simulink model "PCC_Calibration_Simu"  (R2015b)
settings: Solver=ode3  StartTime=0.0  StopTime=1373  FixedStep=0.01  RelTol=1e-3
model workspace: external: MAT-File params.mat (data not in the file)
undefined symbols (not defined in the file): aeroDragCoeff, airDensity, discIntervalf, discIntervals, DiscIntNeverNeededParam, FD, frontArea, G1, G2, G3, G4, G5, G6, gravity, inertialMassVeh, iterNum, lambdaRange, magnitude, massVeh, MDL, powerWeif, powerWeis, predPeriodf, predPeriods, rollingResistCoeff, terminThreshold, terminTimedis, terminVeloweif, terminVeloweis, wheelRadius, z_ACCe
libraries: simulink x16
(part 3 of 5)

== matlab function PCC_Calibration_Simu/Road_map_information1 ==
  data: u1 input; y1 output; y2 output; y3 output
function [y1,y2,y3] = fcn(u1)
%% _________________________________________________________________________________________________________________________________________________________________外界参数 模拟地图信息，需要单独设立地图接口
dis=u1;%当前距离开始的位置
p_po=[0,-2.27524037800000,-2.26950629100000,-2.87172075000000,-2.27524037800000,-2.88893122700000,-5.48585446200000,-2.26950629100000,-1.43254373800000,-0.567237483000000,-1.43254373800000,-0.584427085000000,-0.561507627000000,0.567237483000000,-0.567237483000000,0.475560430000000,-0.475560430000000,0.475560430000000,-0.567237483000000,0,0.945423264000000,1.70193492400000,0.956883999000000,1.70193492400000,0.945423264000000,1.70193492400000,1.14026128000000,1.76498914100000,1.13453057300000,0.475560430000000,-0.475560430000000,-1.13453057300000,-0.475560430000000,-1.13453057300000,-0.475560430000000,-1.13453057300000,-2.38419243000000,-1.13453057300000,-1.91976780400000,-2.88319437200000,-2.27524037800000,-2.88319437200000,-1.70193492400000,-2.88319437200000,-2.27524037800000,-3.41685336700000,-2.37272339300000,-3.34797844600000,-2.26950629100000,-2.86598398300000,-2.27524037800000,-2.88319437200000,-1.89683677500000,-2.86598398300000,-1.70193492400000,-2.84877385200000,-1.90830225200000,-2.27524037800000,-1.42108102800000,-0.567237483000000,-1.43827511400000,-0.567237483000000,0.475560430000000,1.13453057300000,1.90830225200000,1.13453057300000,1.89683677500000,1.12879987700000,1.90830225200000,1.91976780400000,2.86598398300000,1.93123343400000,3.36519671800000,2.41860011500000,3.38815488800000,1.91976780400000,2.90040502300000,3.82446784900000,2.90040502300000,1.93123343400000,2.88893122700000,1.91403501800000,2.88893122700000,1.93123343400000,0.962614381000000,0,-0.956883999000000,-1.71339917100000,-0.962614381000000,-1.62168707500000,-1.43254373800000,0,-2.26950629100000,-1.42108102800000,-2.37845790000000,-1.70193492400000,-2.38419243000000,-3.33649976600000,-2.40139616400000,-1.69620282600000,-2.40139616400000,-1.13453057300000,-0.481290208000000,-1.12879987700000,-0.475560430000000,-1.32365024300000,0,0.567237483000000,-0.567237483000000,-0.561507627000000,-1.13453057300000,-0.475560430000000,0.567237483000000,-0.956883999000000,0,-1.12879987700000,0,-0.951153627000000,0,1.14026128000000,1.90830225200000,2.84303719900000,1.90256950400000,2.86024724400000,1.90830225200000,2.38992698400000,1.70766703900000,2.38992698400000,2.27524037800000,3.37093621000000,2.37845790000000,3.35945726000000,2.38992698400000,2.27524037800000,2.87172075000000,2.28097448800000,3.32502122000000,2.40139616400000,2.26950629100000,3.42259316500000,2.37272339300000,3.42259316500000,2.83730057400000,2.82009087100000,3.42259316500000,2.28097448800000,1.14026128000000,0,-1.14026128000000,-1.91403501800000,-1.14026128000000,-1.90830225200000,-2.84877385200000,-2.26950629100000,-2.84877385200000,-2.09749399500000,-2.28097448800000,-3.42259316500000,-2.28097448800000,-3.42259316500000,-2.83730057400000,-3.42259316500000,-2.28097448800000,-3.51443465800000,-2.83730057400000,-1.91403501800000,-2.38992698400000,-1.70766703900000,-2.40713079000000,-2.40139616400000,-1.66181059200000,-1.69047074500000,-2.84877385200000,-1.91403501800000,-1.69047074500000,-2.84877385200000,-2.21216666100000,-2.84877385200000,-2.28097448800000,-1.43827511400000,-2.28097448800000,-1.43827511400000,-2.28097448800000,-1.14026128000000,0,1.14026128000000,1.91976780400000,3.38241529500000,1.92550061000000,2.38419243000000,0.956883999000000,2.41286544000000,1.44400650500000;];
s_po=[0,0.1,20.8100000000000,58.9100000000000,66.0700000000000,67.0700000000000,70.6600000000000,86.9400000000000,116.910000000000,130.660000000000,131.660000000000,145.430000000000,169.160000000000,178.170000000000,179.160000000000,181.360000000000,183.560000000000,185.970000000000,187.150000000000,223.630000000000,253.830000000000,269.630000000000,270.640000000000,275.230000000000,276.220000000000,278.620000000000,284.150000000000,290.560000000000,290.880000000000,309.290000000000,321.680000000000,328.680000000000,329.700000000000,332.080000000000,333.080000000000,337.880000000000,342.290000000000,343.480000000000,344.490000000000,354.290000000000,355.480000000000,357.480000000000,358.680000000000,360.690000000000,363.080000000000,364.070000000000,367.270000000000,368.480000000000,370.870000000000,371.890000000000,373.070000000000,374.080000000000,391.060000000000,394.660000000000,397.060000000000,399.060000000000,401.460000000000,404.890000000000,412.690000000000,422.090000000000,428.700000000000,429.900000000000,445.490000000000,462.270000000000,476.060000000000,477.270000000000,481.670000000000,484.050000000000,485.060000000000,492.870000000000,497.630000000000,503.570000000000,504.740000000000,507.110000000000,516.600000000000,518.970000000000,521.350000000000,523.710000000000,524.910000000000,581.830000000000,583,586.550000000000,592.490000000000,594.860000000000,611.450000000000,626.670000000000,636.160000000000,645.450000000000,646.450000000000,658.300000000000,659,664.950000000000,665.150000000000,668.550000000000,669.750000000000,684.340000000000,685.330000000000,690.130000000000,712.520000000000,754.060000000000,755.070000000000,756.260000000000,780.100000000000,786.060000000000,787.070000000000,800.040000000000,809.830000000000,839.110000000000,876.190000000000,891.560000000000,944.750000000000,948.150000000000,963.550000000000,964.550000000000,965.740000000000,979.320000000000,980.330000000000,982.530000000000,983.740000000000,1066.69000000000,1082.10000000000,1137.25000000000,1138.26000000000,1182.03000000000,1183.23000000000,1231.42000000000,1257.23000000000,1258.23000000000,1287.74000000000,1289.95000000000,1299.45000000000,1303.04000000000,1307.60000000000,1322.77000000000,1392.04000000000,1394.24000000000,1395.24000000000,1396.46000000000,1429.25000000000,1430.27000000000,1431.27000000000,1433.66000000000,1434.66000000000,1448.46000000000,1466.27000000000,1474.05000000000,1487.66000000000,1504.45000000000,1518.26000000000,1519.25000000000,1527.04000000000,1528.06000000000,1543.64000000000,1558.26000000000,1559.27000000000,1624.84000000000,1635,1636,1640.20000000000,1641.20000000000,1653.79000000000,1659.41000000000,1693.98000000000,1694.98000000000,1708.79000000000,1767.79000000000,1800.96000000000,1802.15000000000,1803.16000000000,1849.82000000000,1894.81000000000,1905.76000000000,1906.77000000000,1919.56000000000,1956.16000000000,1957.17000000000,1971.36000000000,1972.39000000000,1984.68000000000,1994.08000000000,1996.28000000000,1997.28000000000,1999.48000000000,2007.88000000000,2022.86000000000,2047.98000000000,2098.71000000000,2105.85000000000,2109.41000000000,2142.55000000000,2147.31000000000,2153.24000000000,2155.59000000000;];
S_po=[s_po';s_po'+max(s_po)+0.01;0.01+s_po'+max(0.01+s_po'+max(s_po))];
% P_po=[p_po';p_po';p_po'];
P_po=[0;0;0;0;-0.237780215000000;-0.237780215000000;-0.237780215000000;-0.237780215000000;-0.237780215000000;-0.237780215000000;-0.237780215000000;-0.237780215000000;-0.237780215000000;-0.237780215000000;-0.237780215000000;-0.237780215000000;-0.475560430000000;-0.475560430000000;-0.475560430000000;-0.475560430000000;-0.475560430000000;-0.475560430000000;-0.475560430000000;-0.475560430000000;-0.475560430000000;-0.475560430000000;-0.475560430000000;-0.475560430000000;-0.475560430000000;-0.475560430000000;-0.475560430000000;-0.475560430000000;-0.521398956500000;-0.850884028000000;-1.13453057300000;-1.13453057300000;-1.13453057300000;-1.41823274850000;-1.79938584950000;-1.90830228950000;-1.90830228950000;-2.09463704750000;-2.09463704750000;-2.27237333450000;-2.27237333450000;-2.27237333450000;-2.27237333450000;-2.27237333450000;-2.27237333450000;-2.27237333450000;-2.27237333450000;-2.27237333450000;-2.09463704750000;-2.09463704750000;-2.08890427150000;-1.90256951350000;-1.79938584950000;-1.70193492400000;-1.57010501900000;-1.42967807100000;-0.994159255500000;-0.567237483000000;-0.0458385265000000;0.802180153500000;1.13166522500000;1.13453057300000;1.51568367400000;1.90256951350000;1.90830225200000;1.91116863500000;1.91116863500000;1.91116863500000;1.91116863500000;1.91116863500000;1.91116863500000;1.91116863500000;1.91116863500000;1.91116863500000;1.91116863500000;1.91116863500000;1.91116863500000;1.91116863500000;1.91116863500000;1.91116863500000;1.43832469950000;0.481307190500000;0;-0.478441999500000;-0.719087103500000;-0.959749190000000;-0.959749190000000;-1.04570712900000;-1.04570712900000;-1.04570712900000;-1.04570712900000;-1.04570712900000;-1.13166522500000;-1.13166522500000;-1.13166522500000;-1.13166522500000;-1.13166522500000;-1.13166522500000;-1.13166522500000;-1.12879987700000;-1.12879987700000;-1.04284193800000;-0.954018813000000;-0.954018813000000;-0.759195555000000;-0.564372555000000;-0.521398917500000;-0.478425319000000;-0.475560430000000;-0.237780215000000;0;0;0;0.283618741500000;0.567237483000000;0.853749381500000;1.42396415950000;1.80511827150000;1.90543587800000;1.90830225200000;2.08890427150000;2.27237333450000;2.27524037800000;2.27810743300000;2.32684894050000;2.37559064650000;2.38419244200000;2.38419244200000;2.38419244200000;2.38419244200000;2.38419244200000;2.38419244200000;2.38419244200000;2.37559064650000;2.37559064650000;2.32684894050000;2.32684894050000;2.28097448800000;2.28097448800000;2.27810743300000;2.27810743300000;2.27237333450000;1.70488378550000;0.570130640000000;-0.570130640000000;-1.14026128000000;-1.52428176600000;-1.91116863500000;-1.91403501800000;-1.91403501800000;-2.00576450650000;-2.18350014300000;-2.18350014300000;-2.18350014300000;-2.27524038950000;-2.27524038950000;-2.27524038950000;-2.28097448800000;-2.28097448800000;-2.28097448800000;-2.28097448800000;-2.28097448800000;-2.28097448800000;-2.28097448800000;-2.28097448800000;-2.28097448800000;-2.28097448800000;-2.28097448800000;-2.28097448800000;-2.28097448800000;-2.24657057450000;-2.06310083950000;-1.91403501800000;-1.81085102850000;-1.69906889200000;-1.69047074500000;-1.69047074500000;-1.69047074500000;-1.69047074500000;-1.69047074500000;-1.69047074500000;-1.69047074500000;-1.80225288150000;-1.80225288150000;-1.56437292950000;-1.43827511400000;-1.43540942600000;-1.43254373800000;-1.28640250900000;-0.862344182500000;-0.575832284000000;-0.567237483000000;-0.564372555000000;-0.564372555000000;-0.518534028500000;-0.237780215000000;-0.237780215000000;-0.237780215000000;-0.237780215000000;-0.237780215000000;-0.237780215000000;-0.237780215000000;-0.237780215000000;-0.237780215000000;-0.237780215000000;-0.475560430000000;-0.475560430000000;-0.475560430000000;-0.475560430000000;-0.475560430000000;-0.475560430000000;-0.475560430000000;-0.475560430000000;-0.475560430000000;-0.475560430000000;-0.475560430000000;-0.475560430000000;-0.475560430000000;-0.475560430000000;-0.475560430000000;-0.475560430000000;-0.521398956500000;-0.850884028000000;-1.13453057300000;-1.13453057300000;-1.13453057300000;-1.41823274850000;-1.79938584950000;-1.90830228950000;-1.90830228950000;-2.09463704750000;-2.09463704750000;-2.27237333450000;-2.27237333450000;-2.27237333450000;-2.27237333450000;-2.27237333450000;-2.27237333450000;-2.27237333450000;-2.27237333450000;-2.27237333450000;-2.09463704750000;-2.09463704750000;-2.08890427150000;-1.90256951350000;-1.79938584950000;-1.70193492400000;-1.57010501900000;-1.42967807100000;-0.994159255500000;-0.567237483000000;-0.0458385265000000;0.802180153500000;1.13166522500000;1.13453057300000;1.51568367400000;1.90256951350000;1.90830225200000;1.91116863500000;1.91116863500000;1.91116863500000;1.91116863500000;1.91116863500000;1.91116863500000;1.91116863500000;1.91116863500000;1.91116863500000;1.91116863500000;1.91116863500000;1.91116863500000;1.91116863500000;1.91116863500000;1.91116863500000;1.43832469950000;0.481307190500000;0;-0.478441999500000;-0.719087103500000;-0.959749190000000;-0.959749190000000;-1.04570712900000;-1.04570712900000;-1.04570712900000;-1.04570712900000;-1.04570712900000;-1.13166522500000;-1.13166522500000;-1.13166522500000;-1.13166522500000;-1.13166522500000;-1.13166522500000;-1.13166522500000;-1.12879987700000;-1.12879987700000;-1.04284193800000;-0.954018813000000;-0.954018813000000;-0.759195555000000;-0.564372555000000;-0.521398917500000;-0.478425319000000;-0.475560430000000;-0.237780215000000;0;0;0;0.283618741500000;0.567237483000000;0.853749381500000;1.42396415950000;1.80511827150000;1.90543587800000;1.90830225200000;2.08890427150000;2.27237333450000;2.27524037800000;2.27810743300000;2.32684894050000;2.37559064650000;2.38419244200000;2.38419244200000;2.38419244200000;2.38419244200000;2.38419244200000;2.38419244200000;2.38419244200000;2.37559064650000;2.37559064650000;2.32684894050000;2.32684894050000;2.28097448800000;2.28097448800000;2.27810743300000;2.27810743300000;2.27237333450000;1.70488378550000;0.570130640000000;-0.570130640000000;-1.14026128000000;-1.52428176600000;-1.91116863500000;-1.91403501800000;-1.91403501800000;-2.00576450650000;-2.18350014300000;-2.18350014300000;-2.18350014300000;-2.27524038950000;-2.27524038950000;-2.27524038950000;-2.28097448800000;-2.28097448800000;-2.28097448800000;-2.28097448800000;-2.28097448800000;-2.28097448800000;-2.28097448800000;-2.28097448800000;-2.28097448800000;-2.28097448800000;-2.28097448800000;-2.28097448800000;-2.28097448800000;-2.24657057450000;-2.06310083950000;-1.91403501800000;-1.81085102850000;-1.69906889200000;-1.69047074500000;-1.69047074500000;-1.69047074500000;-1.69047074500000;-1.69047074500000;-1.69047074500000;-1.69047074500000;-1.80225288150000;-1.80225288150000;-1.56437292950000;-1.43827511400000;-1.43540942600000;-1.43254373800000;-1.28640250900000;-0.862344182500000;-0.575832284000000;-0.567237483000000;-0.564372555000000;-0.564372555000000;-0.518534028500000;-0.237780215000000;-0.237780215000000;-0.237780215000000;-0.237780215000000;-0.237780215000000;-0.237780215000000;-0.237780215000000;-0.237780215000000;-0.237780215000000;-0.237780215000000;-0.475560430000000;-0.475560430000000;-0.475560430000000;-0.475560430000000;-0.475560430000000;-0.475560430000000;-0.475560430000000;-0.475560430000000;-0.475560430000000;-0.475560430000000;-0.475560430000000;-0.475560430000000;-0.475560430000000;-0.475560430000000;-0.475560430000000;-0.475560430000000;-0.521398956500000;-0.850884028000000;-1.13453057300000;-1.13453057300000;-1.13453057300000;-1.41823274850000;-1.79938584950000;-1.90830228950000;-1.90830228950000;-2.09463704750000;-2.09463704750000;-2.27237333450000;-2.27237333450000;-2.27237333450000;-2.27237333450000;-2.27237333450000;-2.27237333450000;-2.27237333450000;-2.27237333450000;-2.27237333450000;-2.09463704750000;-2.09463704750000;-2.08890427150000;-1.90256951350000;-1.79938584950000;-1.70193492400000;-1.57010501900000;-1.42967807100000;-0.994159255500000;-0.567237483000000;-0.0458385265000000;0.802180153500000;1.13166522500000;1.13453057300000;1.51568367400000;1.90256951350000;1.90830225200000;1.91116863500000;1.91116863500000;1.91116863500000;1.91116863500000;1.91116863500000;1.91116863500000;1.91116863500000;1.91116863500000;1.91116863500000;1.91116863500000;1.91116863500000;1.91116863500000;1.91116863500000;1.91116863500000;1.91116863500000;1.43832469950000;0.481307190500000;0;-0.478441999500000;-0.719087103500000;-0.959749190000000;-0.959749190000000;-1.04570712900000;-1.04570712900000;-1.04570712900000;-1.04570712900000;-1.04570712900000;-1.13166522500000;-1.13166522500000;-1.13166522500000;-1.13166522500000;-1.13166522500000;-1.13166522500000;-1.13166522500000;-1.12879987700000;-1.12879987700000;-1.04284193800000;-0.954018813000000;-0.954018813000000;-0.759195555000000;-0.564372555000000;-0.521398917500000;-0.478425319000000;-0.475560430000000;-0.237780215000000;0;0;0;0.283618741500000;0.567237483000000;0.853749381500000;1.42396415950000;1.80511827150000;1.90543587800000;1.90830225200000;2.08890427150000;2.27237333450000;2.27524037800000;2.27810743300000;2.32684894050000;2.37559064650000;2.38419244200000;2.38419244200000;2.38419244200000;2.38419244200000;2.38419244200000;2.38419244200000;2.38419244200000;2.37559064650000;2.37559064650000;2.32684894050000;2.32684894050000;2.28097448800000;2.28097448800000;2.27810743300000;2.27810743300000;2.27237333450000;1.70488378550000;0.570130640000000;-0.570130640000000;-1.14026128000000;-1.52428176600000;-1.91116863500000;-1.91403501800000;-1.91403501800000;-2.00576450650000;-2.18350014300000;-2.18350014300000;-2.18350014300000;-2.27524038950000;-2.27524038950000;-2.27524038950000;-2.28097448800000;-2.28097448800000;-2.28097448800000;-2.28097448800000;-2.28097448800000;-2.28097448800000;-2.28097448800000;-2.28097448800000;-2.28097448800000;-2.28097448800000;-2.28097448800000;-2.28097448800000;-2.28097448800000;-2.24657057450000;-2.06310083950000;-1.91403501800000;-1.81085102850000;-1.69906889200000;-1.69047074500000;-1.67614066850000;-1.55004285300000;-1.43827511400000;-1.28926819700000;-0.570130640000000;0;0;0;0;0;0;0;0];
Po_s=size(P_po);
A_a=[0,600,601,800,801,1000,1001,120000]';%三百个点，每个点1m，301行1列
B_a2=[0,0,2,2,-2,-2,0,0]';
B_a1=[0,0,0,0,0,0,0,0]';
% ii=1;
% for i=1:301
%     for mi=ii:Po_s(1)
%         if((dis+i-1)>=S_po(mi)&&(dis+i-1)<S_po(mi+1))
%             B_a(i)=P_po(mi);
%             ii=mi;
%             break;
%         end
%     end
% end
C_a=ones(8,1)*30;%限速信息
% if(dis<800)
%     B_a=B_a1;
% else
%     B_a=B_a2;
% end
y1=A_a;
y2=B_a2;
y3=C_a;

== matlab function PCC_Calibration_Simu/host vehicle/Enabled Subsystem1/MATLAB Function ==
  data: u1 input; y1 output; y2 output; u2 input; u3 input; u4 input; u5 input; u6 input; u7 input; u8 input; u9 input; y3 output; u10 input; u11 input; u12 input; u13 input; u14 input; u15 input; u16 input; u17 input; u18 input; u19 input; u20 input; u21 input; u22 input; u23 input; u24 input; u25 input; u26 input; u27 input
function [y1,y2,y3] = fcn(u1,u2,u3,u4,u5,u6,u7,u8,u9,u10,u11,u12,u13,u14,u15,u16,u17,u18,u19,u20,u21,u22,u23,u24,u25,u26,u27)
%#codegen
%************************************************************************************************%以下为优化控制
Delta=u11;%离散化
Ne=u1;
Vh=u2;
Vr=u3*1.05;%期望车速
Te_u0=u4;
ig0=u5;%当前时刻挡位
dis=u6;
S_po=u7;%当前距离开始的距离向量，预留位置
P_po=u8;%当前距离开始的坡度向量
tim=u9;
tf=u10;%预测时间15s
wr=u12;%终端速度权重
mm=u13;%动力性权重
Na=301;
ii=0;

if(tim==fix(tim/0.01)*0.01)
    
    
    
    
    
    
    
%% 车辆固有参数
cd=u17;%风阻系数
Af=u18;%有效迎风面积
ro=1.205;%空气密度
M=u19;%整车质量
af=cd*Af*ro/2/M;%风阻参数
f=0.011;%滚动阻力系数
g=9.8;%重力加速度
itat=0.94;%机械效率
rw=u20/1000;%车轮半径
% p2=3.02907665419964E-5;%发动机油耗拟合参数
% p3=4.27560640521964E-8;
% p4=-0.00271052610070109;
% p5=5.93301576094487E-6;
% p6=-2.0545387116593E-10;
% p7=4.68494877338369E-5;
% p8=-2.63343173129148E-8;
% p9=6.91834817840693E-12;
p1=-0.0221169655141491;
p2=0.000216402696874227;
p3=5.21621452533686E-9;
p4=-0.00171519706716103;
p5=5.36124098434418E-6;
p6=-2.79120978391711E-10;
p7=3.88461733908615E-5;
p8=-1.96505868079643E-8;
p9=6.89898750358085E-12;%在发动机转速3000转内拟合，没有数据的部分作何延伸。
k2=p2*30/pi/rw;%公式推导过程参数转换
k3=p3*(30/pi/rw)^2;
k4=p4;
k5=p5*30/pi/rw;
k6=p6*(30/pi/rw)^2;
k7=p7;
k8=p8*30/pi/rw;
k9=p9*(30/pi/rw)^2;
Ig=[u21*u22 u21*u23 u21*u24 u21*u25 u21*u26 u21*u27];%变速箱速比
Temax=[161.31,170.09,177.38,184.31,192.35,200.13,200.53,199.15,198.72,203.47,211.59,207.43,212.7,215.05,212.68,210.91,206.09,202.94,198.51,197.64,191.85,187.34,185.62,172.03]*0.8;%经济性驾驶规定最大行驶力矩
Nemax=[800,1251,1500,1750,2000,2250,2500,2750,3000,3250,3500,3750,4000,4149,4250,4500,4750,5000,5250,5501,5750,5876,6000,6250];%最大行驶力矩对应的转速
if(Ne<=800)%保证输入的转速可以进行计算
    Ne=800;
elseif(Ne>=5500)%保证输入的转速可以进行计算
    Ne=5500;
end
temax01=interp1(Nemax,Temax,Ne);%当前可以输出的最大力矩
ig_u=ig0;%初始档位，位置，在加速过程中，可以将换挡信息加进来以保证转矩优化的合理性
lambda_L=-u16;%算法求解参数，初始化二分区间 aa bb aa1 bb1
lambda_U=u16;%算法求解参数，初始化二分区间 aa bb aa1 bb1
Cn=u14;%算法迭代最长次数
%% 计算

Np=round(tf/Delta);%预测时域离散点数
Aa=[4,6,8,10,12,14,16,18,20,40];
Ba=[85,100,110,120,130,140,145,150,150,150];
temax0=interp1(Aa,Ba,Vh,'linear');
if(Vh<=0.5*Vr) %本车速度小于0.4Vr，此时需要加速
    Te=min(temax0,temax01);
elseif(Vh>1.2*Vr) %本车速度大于1.2Vr，此时需要滑行
    Te=0;
else
%******************************************************************************************************************************************************求解优化问题
s=dis;
v=Vh;%初始速度
lambda=lambda_L;
ii_po=1;
for j=1:Np
    A1=k7+k8*Ig(ig_u)*v+k9*Ig(ig_u)^2*v^2;  %H=A1*Tm^2+B1*Tm
    B1=k4+k5*Ig(ig_u)*v+k6*Ig(ig_u)^2*v^2+lambda*Ig(ig_u)*itat/M/rw;
    if(A1>0)
        if(-B1/2/A1<=0)
            te_u=0;
        elseif(-B1/2/A1>=temax0)
            te_u=temax0;
        else
            te_u=-B1/2/A1;
        end
    elseif(A1<0)
        if(-B1/2/A1<=1/2*temax0)
            te_u=temax0;
        else
            te_u=0;
        end
    else
        if(B1>=0)
            te_u=0;
        else
            te_u=temax0;
        end
    end
    bk=k2*Ig(ig_u)+2*k3*Ig(ig_u)^2*v+(k5*Ig(ig_u)+2*k6*Ig(ig_u)^2*v)*te_u+(k8*Ig(ig_u)+2*k9*Ig(ig_u)^2*v)*te_u^2+2*wr*(v-Vr);
    lambda=lambda+Delta*(2*af*v*lambda-bk);

    po=0;
%     for i_po=ii_po:Na-1
%         if(s>=S_po(i_po)&&s<S_po(i_po+1))
%             po=P_po(i_po);
%             ii_po=i_po;
%             break
%         end
%     end
    po=interp1(S_po,P_po,s,'linear');
    ar=f*g*cos(po/180*pi);%滚动阻力加速度
    ag=g*sin(po/180*pi);%坡度阻力加速度
    v=v+Delta*(te_u*Ig(ig_u)*itat/M/rw-ar-ag-af*v^2); %或得下一时刻的预测车速
    if(v<=0)
        v=0;
    end
    s=s+v*Delta;
end
aa=lambda_L;
bb=lambda_U;
aa1=lambda-mm*(v-Vr);
Te_u1=0;
Te_u2=0;
for ii=1:Cn
    s=dis;
    v=Vh;%初始速度
    lambda=aa+0.5*(bb-aa);
    ii_po=1;
    for j=1:Np
        A1=k7+k8*Ig(ig_u)*v+k9*Ig(ig_u)^2*v^2;  %H=A1*Tm^2+B1*Tm
        B1=k4+k5*Ig(ig_u)*v+k6*Ig(ig_u)^2*v^2+lambda*Ig(ig_u)*itat/M/rw;
        if(A1>0)
            if(-B1/2/A1<=0)
                te_u=0;
            elseif(-B1/2/A1>=temax0)
                te_u=temax0;
            else
                te_u=-B1/2/A1;
            end
        elseif(A1<0)
            if(-B1/2/A1<=1/2*temax0)
                te_u=temax0;
            else
                te_u=0;
            end
        else
            if(B1>=0)
                te_u=0;
            else
                te_u=temax0;
            end
        end
        if(j==1)
            Te_u1=te_u;
        end
        if(j==2)
            Te_u2=te_u;
        end
        bk=k2*Ig(ig_u)+2*k3*Ig(ig_u)^2*v+(k5*Ig(ig_u)+2*k6*Ig(ig_u)^2*v)*te_u+(k8*Ig(ig_u)+2*k9*Ig(ig_u)^2*v)*te_u^2+2*wr*(v-Vr);
        lambda=lambda+Delta*(2*af*v*lambda-bk);
        
        po=0;
%         for i_po=ii_po:Na-1
%             if(s>=S_po(i_po)&&s<S_po(i_po+1))
%                 po=P_po(i_po);
%                 ii_po=i_po;
%                 break
%             end
%         end
        po=interp1(S_po,P_po,s,'linear');
        ar=f*g*cos(po/180*pi);%滚动阻力加速度
        ag=g*sin(po/180*pi);%坡度阻力加速度
        v=v+Delta*(te_u*Ig(ig_u)*itat/M/rw-ar-ag-af*v^2); %或得下一时刻的预测车速
        if(v<=0)
            v=0;
        end
        s=s+v*Delta;
    end
    if(abs(lambda-mm*(v-Vr))<0.02)
        break;
    else
        if(aa1*(lambda-mm*(v-Vr))<=0)%判断跨越零点位置
            bb=aa+0.5*(bb-aa);
        else
            aa=aa+0.5*(bb-aa);
            aa1=lambda;
        end
    end
end
if(abs(lambda-mm*(v-Vr))<u15)%证明计算出结果
    Te_u=(Te_u1+Te_u2)/2;
    if(Te_u<=5)
        Te_u=0;
    end
else
    Te_u=Te_u0;
end
Te=Te_u;
end
%% 输出结果

else
   Te=Te_u0;
end

Te=min(150,Te);
y1=Te;
y2=0;
y3=ii;

== matlab function PCC_Calibration_Simu/host vehicle/Enabled Subsystem3/MATLAB Function ==
  data: u1 input; y1 output; u2 input; u3 input; u4 input; y2 output; u5 input; u6 input; u7 input; y3 output
function [y1,y2,y3]= fcn(u1,u2,u3,u4,u5,u6,u7)
%#codegen
uu=u1;%后续会用到
Vp=u2;
Vh=u3;
bon=u4;
Mode=u5;
uu_lim_0=u6;
Vh0=u7;
if(Mode==4)
    uu_lim=uu_lim_0;
    vv=Vh0;
else
    uu_lim=uu;
    vv=Vh;
end
if(vv>=60/3.6)
    br_acc=[5,3,2.8,2.8,0.7,0];
elseif(vv>=50/3.6)
    br_acc=[5,3,2.8,2.8,0.65,0];
elseif(vv>=40/3.6)
    br_acc=[5,3,2.8,2.8,0.6,0];
elseif(vv>=30/3.6)
    br_acc=[4,2.5,2,2,0.55,0];
else
    br_acc=[4,2,1.5,1,0.5,0];
end
br_uu=[0,0.2*uu_lim,uu_lim*0.25,uu_lim*0.7,uu_lim,2];%保证一般的最大制动力维持在2.5
if(uu>=uu_lim)
    uu=uu_lim;
end
br=interp1(br_uu,br_acc,uu,'linear');
if(br<0.05)
    br=0;
end
%***********************************************************************************************%控制量
%% 输出结果
y1=br;
y2=uu_lim;
y3=vv;

== matlab function PCC_Calibration_Simu/host vehicle/Enabled Subsystem4/MATLAB Function ==
  data: u1 input; y1 output; u2 input; u3 input; y2 output; u4 input; y3 output; u5 input; y4 output; u6 input
function [y1,y2,y3,y4]= fcn(u1,u2,u3,u4,u5,u6)
%#codegen
dis=u1;
Vh=u2;
Vp=u3;
dV=Vp-Vh;
Mod=u4;
br0=u5;
uu0=u6;
uu=5;
if(dV>=0.5||(dV>=-0.5&&Mod==1))
    mode=1;
    if(Vp-Vh>=3)
        A1=[0 4 6 6.001 8 15 25 2000];
        B1=[0 0 0 20 40 60 60 60];
    elseif(Vp-Vh>=2)
        A1=[0 4 6 6.001 8 15 25 2000];
        B1=[0 0 0 20 30 50 60 60];
    else
        A1=[0 4 6 6.001 8 15 25 2000];
        B1=[0 0 0 10 20 40 60 60];
    end
    C_1=[0 4 6 6.001 8 15 25 2000];
    C1=[0.5 0.5 0.25 0 0 0 0 0];
    Te=interp1(A1,B1,dis,'linear');
    br=interp1(C_1,C1,dis,'linear');
    if(br<=0.25)
        br=0;
    end
else       
    mode=2;
    if(Vh<=0.25&&dis<=10)
        br=1;
    elseif(Vh<=0.25&&dis>10)
        br=0;
    else
        Aa=[0.1,0.5,1,2,3,4,5,6];%速度
        Ba= [2,3,4,6,9,11,13,15]+0.5;
        if(br0<=0.2||uu0==0)%上一时刻没有制动或者不在这一区域
            uu=interp1(Aa,Ba,Vh,'linear');%开始制动的
        else
            uu=uu0;
        end
        Br_tic=[0,0.2*uu,0.45*uu,uu,uu+0.001,30];%制动力对应
        Br=[2,1.5,1,0.5,0,0];%制动力
        if(dis>=30)
            br=0;
        else
            br=interp1(Br_tic,Br,dis,'linear');
        end   
    end
    t1=[0 15 15.1 20 25 2000];
    t2=[0 0 10 20 60 60];
    Te=interp1(t1,t2,dis,'linear');
    if(Te>=1)
        br=0;
    end
end
%***********************************************************************************************%控制量
%% 输出结果
y1=Te;
y2=br;
y3=mode;
y4=uu;

== matlab function PCC_Calibration_Simu/host vehicle/Enabled Subsystem5/MATLAB Function ==
  data: u1 input; y1 output; y2 output; u2 input; u3 input; u4 input; u5 input; u6 input; u7 input; u8 input; u9 input; u10 input; u11 input; u12 input; u13 input; u14 input; u15 input; u16 input; u17 input; u18 input; u19 input; u20 input; u21 input; u22 input; u23 input; u24 input; u25 input; u26 input; u27 input; u28 input; u29 input; u30 input
function [y1,y2] = fcn(u1,u2,u3,u4,u5,u6,u7,u8,u9,u10,u11,u12,u13,u14,u15,u16,u17,u18,u19,u20,u21,u22,u23,u24,u25,u26,u27,u28,u29,u30)
%#codegen
%************************************************************************************************%以下为优化控制
dV=u1;%后续会用到
dS=u2;
Ne=u3;
Vh=u4;
Te0=u5;
Vr=u6;%期望车速
ig0=u7;%当前时刻挡位
tim=u11;
ii=0;
if(tim==fix(tim/0.1)*0.1)




%% 外界参数 模拟地图信息，需要单独设立地图接口
dis=u8;%当前距离开始的位置，预留位置
S_po=u9;%当前距离开始的距离向量，预留位置
P_po=u10;%当前距离开始的坡度向量
ap0=0;%当前时刻前车的加速度
if(ap0>=0.5)
    ap0=0.5;
elseif(ap0<=-0.5)
    ap0=-0.5;
end
Na=301;
if(ig0==0)
    Te=0;
else

%% 车辆固有参数
cd=u20;%风阻系数
Af=u21;%有效迎风面积
ro=1.205;%空气密度
M=u22;%整车质量
af=cd*Af*ro/2/M;%风阻参数
f=0.011;%滚动阻力系数
g=9.8;%重力加速度
itat=0.94;%机械效率
rw=u23/1000;%车轮半径
p1=-0.0221169655141491;
p2=0.000216402696874227;
p3=5.21621452533686E-9;
p4=-0.00171519706716103;
p5=5.36124098434418E-6;
p6=-2.79120978391711E-10;
p7=3.88461733908615E-5;
p8=-1.96505868079643E-8;
p9=6.89898750358085E-12;%在发动机转速3000转内拟合，没有数据的部分作何延伸。
k2=p2*30/pi/rw;%公式推导过程参数转换
k3=p3*(30/pi/rw)^2;
k4=p4;
k5=p5*30/pi/rw;
k6=p6*(30/pi/rw)^2;
k7=p7;
k8=p8*30/pi/rw;
k9=p9*(30/pi/rw)^2;
%Ig=[16.78 9.09 5.92 4.66 3.66 2.63];%变速箱速比
Ig=[u24*u25 u24*u26 u24*u27 u24*u28 u24*u29 u24*u30];%变速箱速比
Temax=[161.31,170.09,177.38,184.31,192.35,200.13,200.53,199.15,198.72,203.47,211.59,207.43,212.7,215.05,212.68,210.91,206.09,202.94,198.51,197.64,191.85,187.34,185.62,172.03];%经济性驾驶规定最大行驶力矩
Nemax=[800,1251,1500,1750,2000,2250,2500,2750,3000,3250,3500,3750,4000,4149,4250,4500,4750,5000,5250,5501,5750,5876,6000,6250];%最大行驶力矩对应的转速
Temin=0;

% Ca_1=[3 4 6 8 10 12 16 40];%本车速度定义下的的进入制动的开始时距_速度
% Ca_2=[4.6 3.9 3.3 2.8 2.5 2.3 2 1.8]*1.1;%本车速度定义下的进入制动的开始时距
% Dtc=interp1(Ca_1,Ca_2,Vh,'linear')*1.1;
% Dtc=3.5;
%***********************************************************************************************************************************
%% 控制器参数，需调整
beta1=0.5;%前车速度预测参数
gama1=5;%前车速度预测参数
beta2=0.5;%前车速度预测参数
gama2=40;%前车速度预测参数
ap0=0;
Delta = u13;%离散化
Dtc = u14;%终端时距
Cn=u17;%算法迭代最长次数
if(Ne<=800)%保证输入的转速可以进行计算
    Ne=800;
elseif(Ne>=5500)%保证输入的转速可以进行计算
    Ne=5500;
end
Aa=[4,6,8,10,12,14,16,18,20,40];
Ba=[85,100,110,120,130,140,145,150,150,150];
zeta1=interp1(Aa,Ba,Vh,'linear');
zeta2=interp1(Nemax,Temax,Ne,'linear');%当前可以输出的最大力矩
temax0=min(zeta1,zeta2);
ig_u=ig0;%初始档位，位置，在加速过程中，可以将换挡信息加进来以保证转矩优化的合理性
lambda_L=-u19;%算法求解参数，初始化二分区间 aa bb aa1 bb1
lambda_U=u19;%算法求解参数，初始化二分区间 aa bb aa1 bb1
%% 计算
tf=u12;%预测时间8s
wr=u16;%动力性权重
mm=u15;%终端速度权重
Termination = u18;
Np=round(tf/Delta);%预测时域离散点数
%***********************************************************************************************************************************预测前车在未来一段时间的速度和位移
sp0=dS;%当前时刻前车的位移，设定本车当前时刻的位移是0
vp0=dV+Vh;%当前时刻前车的速度
% coder.varsize('vp', [1024 1]); %n must never exceed 1024
% coder.varsize('ap', [1024 1]); %n must never exceed 1024
% coder.varsize('sp', [1024 1]); %n must never exceed 1024
vp=zeros(1024,1);%预测时域内前车速度
ap=zeros(1024,1);%预测时域内前车加速度
sp=zeros(1024,1);%预测时域内前车位移
vp(1)=vp0;
ap(1)=ap0;
sp(1)=sp0;
for j=1:Np
    if(ap0<=0)%预测模型
        ap(j)=ap0/(1+exp(-1*beta1*(vp(j)-gama1)));
    else
        ap(j)=ap0/(1+exp(beta2*(vp(j)-gama2)));
    end
    vp(j+1)=vp(j)+Delta*ap(j);
    if(vp(j+1)<=0)
        vp(j+1)=0;
    end
    sp(j+1)=sp(j)+Delta*vp(j);
end
%*******************************************************************************************************************************************************%计算终端条件
Vmax1=(sp(Np+1)-0.5*tf*Vh)/(Dtc+0.5*tf);
Vn=min(Vr,Vmax1);
vr=Vn;
%******************************************************************************************************************************************************求解优化问题
s=dis;
v=Vh;%初始速度
lambda=lambda_L;
ii_po=1;
for j=1:Np
    A1=k7+k8*Ig(ig_u)*v+k9*Ig(ig_u)^2*v^2;  %H=A1*Tm^2+B1*Tm
    B1=k4+k5*Ig(ig_u)*v+k6*Ig(ig_u)^2*v^2+lambda*Ig(ig_u)*itat/M/rw;
    if(A1>0)
        if(-B1/2/A1<=0)
            te_u=Temin;
        elseif(-B1/2/A1>=temax0)
            te_u=temax0;
        else
            te_u=-B1/2/A1;
        end
    elseif(A1<0)
        if(-B1/2/A1<=1/2*temax0)
            te_u=temax0;
        else
            te_u=Temin;
        end
    else
        if(B1>=0)
            te_u=Temin;
        else
            te_u=temax0;
        end
    end
    bk=k2*Ig(ig_u)+2*k3*Ig(ig_u)^2*v+(k5*Ig(ig_u)+2*k6*Ig(ig_u)^2*v)*te_u+(k8*Ig(ig_u)+2*k9*Ig(ig_u)^2*v)*te_u^2+2*wr*(v-vr);
    lambda=lambda+Delta*(2*af*v*lambda-bk);
    po=0;
%     for i_po=ii_po:Na-1
%         if(s>=S_po(i_po)&&s<S_po(i_po+1))
%             po=P_po(i_po);
%             ii_po=i_po;
%             break
%         end
%     end
    po=interp1(S_po,P_po,s,'linear');
    ar=f*g*cos(po/180*pi);%滚动阻力加速度
    ag=g*sin(po/180*pi);%坡度阻力加速度
    v=v+Delta*(te_u*Ig(ig_u)*itat/M/rw-ar-ag-af*v^2); %或得下一时刻的预测车速
    if(v<=0)
        v=0;
    end
    s=s+v*Delta;
end
aa=lambda_L;
bb=lambda_U;
aa1=lambda-mm*(v-Vn);
Te_u1=0;
Te_u2=0;
for ii=1:Cn
    s=dis;
    v=Vh;%初始速度
    lambda=aa+0.5*(bb-aa);
    ii_po=1;
    for j=1:Np
        A1=k7+k8*Ig(ig_u)*v+k9*Ig(ig_u)^2*v^2;  %H=A1*Tm^2+B1*Tm
        B1=k4+k5*Ig(ig_u)*v+k6*Ig(ig_u)^2*v^2+lambda*Ig(ig_u)*itat/M/rw;
        if(A1>0)
            if(-B1/2/A1<=0)
                te_u=Temin;
            elseif(-B1/2/A1>=temax0)
                te_u=temax0;
            else
                te_u=-B1/2/A1;
            end
        elseif(A1<0)
            if(-B1/2/A1<=1/2*temax0)
                te_u=temax0;
            else
                te_u=Temin;
            end
        else
            if(B1>=0)
                te_u=Temin;
            else
                te_u=temax0;
            end
        end
        if(j==1)
            Te_u1=te_u;
        end
        if(j==2)
            Te_u2=te_u;
        end    
        bk=k2*Ig(ig_u)+2*k3*Ig(ig_u)^2*v+(k5*Ig(ig_u)+2*k6*Ig(ig_u)^2*v)*te_u+(k8*Ig(ig_u)+2*k9*Ig(ig_u)^2*v)*te_u^2+2*wr*(v-vr);
        lambda=lambda+Delta*(2*af*v*lambda-bk);
        po=0;
%         for i_po=ii_po:Na-1
%             if(s>=S_po(i_po)&&s<S_po(i_po+1))
%                 po=P_po(i_po);
%                 ii_po=i_po;
%                 break
%             end
%         end
        po=interp1(S_po,P_po,s,'linear');
        ar=f*g*cos(po/180*pi);%滚动阻力加速度
        ag=g*sin(po/180*pi);%坡度阻力加速度
        v=v+Delta*(te_u*Ig(ig_u)*itat/M/rw-ar-ag-af*v^2); %或得下一时刻的预测车速
        if(v<=0)
            v=0;
        end
        s=s+v*Delta;
    end
    if(abs(lambda-mm*(v-Vn))<0.02)
        break;
    else
        if(aa1*(lambda-mm*(v-Vn))<=0)%判断跨越零点位置
            bb=aa+0.5*(bb-aa);
        else
            aa=aa+0.5*(bb-aa);
            aa1=lambda-mm*(v-Vn);
        end
    end
end
if(abs(lambda-mm*(v-Vn))<Termination)%证明计算出结果
    Te_u=(Te_u1+Te_u2)/2;
    if(Te_u<=20)
        Te_u=0;
    end
else
    Te_u=Te0;
end
Te=Te_u;
end



else
    Te=Te0;
end

%% 输出结果
Te=min(Te,150);
y1=Te;
y2=0;

== matlab function PCC_Calibration_Simu/host vehicle/MATLAB Function1 ==
  data: u1 input; y1 output; y2 output; u2 input; u3 input; u4 input; u5 input; y3 output; y4 output; y5 output; u6 input; u7 input; u8 input; y6 output; u9 input; u10 input; u11 input; y7 output
function [y1,y2,y3,y4,y5,y6,y7] = fcn(u1,u2,u3,u4,u5,u6,u7,u8,u9,u10,u11)
%**********************************************************************************************%信号采集
Vh=u1;%本车速度
Vp=u2;%前车速度
dV=Vp-Vh;%前后车速度差
dS=u3;%前后车间距
Scen=u4;%交通情景（前方有车辆、前方无车辆,分别为1,0）
Mode=u5;%当前时刻工作模式
%% 外界参数 模拟地图信息，需要单独设立地图接口
% dis=u9;%当前距离开始的位置，预留位置
% S_po=u10;%当前距离开始的距离向量，预留位置
P_po=u11;%当前距离开始的坡度向量
ca=P_po(1);
%***********************************************************************************************%参数定义  
if(Vh<=4.5&&Mode==0||Vh<=3.5&&Mode~=0)%起步阶段
    model=0;
    uu=1.5;    
    bon=0.3;
    Tc_b=3;
    Tc_bm=0.6;
    Tcmax=5;
else %非起步阶段
%——————————————————————————————————————————————————————待标定参数,确定边界参数
    Aa=[3,5,10,15,20,25,30,35,40];%本车速度定义下的最高限值_速度
    Ba=[14,13,10,7.4,5.5,5,5,5,5]*1.1;%本车速度定义下的进入非跟车模式的时距
    Ca_1=[3 4 6 8 10 12 16 40];%本车速度定义下的的进入制动的开始时距_速度
    Ca_2=[4.6 3.9 3.3 2.8 2.5 2.3 2 1.8]*1.1;%本车速度定义下的进入制动的开始时距
    Value_mode_Tc_b=interp1(Ca_1,Ca_2,Vh,'linear');
    Value_mode_Tc_bm=Value_mode_Tc_b*0.2;
    Value_mode_tcmax=interp1(Aa,Ba,Vh,'linear');
    dS_max1=Vh*Value_mode_tcmax;%计算当前的值
    dS_b1=Vh*Value_mode_Tc_b;
    dS_bm1=Vh*Value_mode_Tc_bm;
    if(dS<=dS_bm1) %如果当前距离小于最小的跟车距离，设定为跟车模式的最小值
        dS=dS_bm1;
    end
    bon1=(dS_b1-dS_bm1)/(dS_max1-dS_bm1);%边界归一化，0-1
    uu1=(dS-dS_bm1)/(dS_max1-dS_bm1);%确定当前在图中的位置，归一化
    if(Mode==1)
        Tcmax=Value_mode_tcmax*0.9;%最高时距
        Tc_b=Value_mode_Tc_b;%开始制动的时距
        Tc_bm=Value_mode_Tc_bm;%制动时距最低值
    else
        if(Mode==4)
            Tc_b=u6;%上一时刻开始制动的时距
            Tc_bm=u7;%上一时刻制动时距最低值
            Tcmax=u8;%最高时距
        else
            Tc_b=Value_mode_Tc_b;%开始制动的时距
            Tc_bm=Value_mode_Tc_bm;%制动时距最低值
            Tcmax=Value_mode_tcmax;%最高时距
        end
    end
    dS_max=Vh*Tcmax;
    dS_b=Vh*Tc_b;
    dS_bm=Vh*Tc_bm;
    if(dS<=dS_bm) %如果当前距离小于最小的跟车距离，设定为跟车模式的最小值
        dS=dS_bm;
    end
    bon=(dS_b-dS_bm)/(dS_max-dS_bm);%边界归一化，0-1
    uu=(dS-dS_bm)/(dS_max-dS_bm);%确定当前在图中的位置，归一化
%***********************************************************************************************%模式判断
    if(dS>=dS_max||Scen==0)
        if(Mode==4&&dV<=-4)
            model=4;%制动
        else
            model=1;%非跟车模式
        end
    else
%模式切换曲线
        L1_v=[-40,-35,-20,-4,-3,0,0.5];
        if(bon+0.6>=1)
            L1_tc=[1,0.999,0.998,bon,bon*0.9,bon*0.8,0];
        elseif(bon+0.9>=1)
            L1_tc=[1,0.999,bon+0.58,bon,bon*0.9,bon*0.8,0];
        else
            L1_tc=[1,bon+0.9,bon+0.6,bon,bon*0.9,bon*0.8,0];
        end
        L2_tc=[1,0.8,(0.8-bon)/4+bon,bon,0];%控制模式切换曲线2
        L2_v=[-4,-4,-2,0,2];
        L3_tc=[1,(bon+1)*0.5,bon*0.5,0];%控制模式切换曲线3
        L3_v=[-4,0,3,5];
        if(uu>=1)
            uu=0.99;
        end
%判断工作模式
        v_bound1=interp1(L1_tc,L1_v,uu,'linear');
        v_bound2=interp1(L2_tc,L2_v,uu,'linear');
        v_bound3=interp1(L3_tc,L3_v,uu,'linear');
        if(dV<=v_bound1||(Mode==4&&dV<=0&&uu<=bon+0.25)||(Mode==4&&dV<=-4)||(Mode==4&&dV<=v_bound1+0.5)||(Mode==4&&dV<=0&&uu1<=bon1+0.3))
            model=4;%制动
        elseif(v_bound1<dV&&dV<=v_bound2)
            model=2;%滑行
        elseif(v_bound2<dV&&dV<=v_bound3)%保持
            if(Mode==3&&dV>=v_bound2+0.5)
                model=3;%加速
            else
                model=2;%滑行
            end
        else
            model=3;%加速
        end
    end
end
%_________________________________________________________________________________________________________________________________________________________________输出结果
y1=model;
y2=uu;%用来确定当前的位置
y3=bon;
y4=Tc_b;
y5=Tc_bm;
y6=Tcmax;
y7=ca;
